simulink model "HydrogenRefuelingStation_Param"  (R2023b)
settings: Solver=VariableStepAuto  StartTime=0.0  StopTime=finSimulation  RelTol=1e-3  AbsTol=1e-3
PreLoadFcn:
  | load hydrogen_properties.mat
  | load silicone_fluid_properties.mat
  | 
  | p_storage = 200; % [bar]
  | p_vehicle_init = 100; % [bar]
  | T_env = 25; % [degC]
  | T_fluid = -60; % [degC]
  | 
  | V_vehicle = 172; % [l]
  | 
  | tube_D = 0.04; % [m]
  | hose_D = 0.0064; % [m]
  | pipe_D = 0.1; % [m]
  | 
  | num_buffer = 2;
  | 
  | intercooler_num_tubes = 25;
  | intercooler_tube_D = 0.008; % [m]
  | intercooler_shell_D = 0.1; % [m]
  | intercooler_L = 2; % [m]
  | 
  | precooler_tube_W = 0.001; % [m]
  | precooler_num_tubes = 50*25;
  | precooler_L = 1; % [m]
values from neighbouring files (symbols this model uses):
  EngDemandTime = 3000    [launch.m]
  EngThrottle = 1    [launch.m]
  ext_bufferEng_D = 0.025    [System_Parameters.m]
  ext_Manifold_D = 0.007    [System_Parameters.m]
  ext_vehTank_D = 0.25    [System_Parameters.m]
  in_bufferEng_D = 0.0064    [System_Parameters.m]
  in_Eng_D = 0.0064    [System_Parameters.m]
  in_Man_D = 0.0064    [System_Parameters.m]
  inOut_vehTank_D = 0.0064    [System_Parameters.m]
  int_bufferEng_D = 0.024    [System_Parameters.m]
  int_Manifold_D = 0.0064    [System_Parameters.m]
  int_vehTank_D = 0.22    [System_Parameters.m]
  L_bufferEng = 1    [System_Parameters.m]
  L_Manifold = 1    [System_Parameters.m]
  L_vehTank = 2    [System_Parameters.m]
  MV_D = 0.0064    [System_Parameters.m]
  out_bufferEng_D = 0.0064/2    (= 0.0032)    [System_Parameters.m]
  out_Eng_D = 0.0064    [System_Parameters.m]
  out_Man_D = 0.0064    [System_Parameters.m]
  Pipe_ConnMan_D = 0.0064    [System_Parameters.m]
  Pipe_ManPR_D = 0.0064    [System_Parameters.m]
  Pipe_ManTank_D = 0.0064    [System_Parameters.m]
  Pipe_PRBuffer_D = 0.0064    [System_Parameters.m]
  redn_PR_D = 0.0064    [System_Parameters.m]
  redn_PR_setP = 160    [System_Parameters.m]
  relief_PR_D = 0.0064    [System_Parameters.m]
  relief_vehTank_D = 0.0064    [System_Parameters.m]
  silicone_fluid =     [silicone_fluid_properties.mat]
  statConn_D = 0.0064    [System_Parameters.m]
  stationTrigger_Time = 2400    [System_Parameters.m]
  SV_D = 0.0064    [System_Parameters.m]
  tank_Man_D = 0.0064    [System_Parameters.m]
  TempCont_vehTank_D = 0.0064    [System_Parameters.m]
  vehConn_D = 0.0064    [System_Parameters.m]
  WP_high = 700    [System_Parameters.m]
libraries: fl_lib x128, nesl_utility x60, SimscapeFluids_lib x41, slpidlib x4
(part 4 of 6)

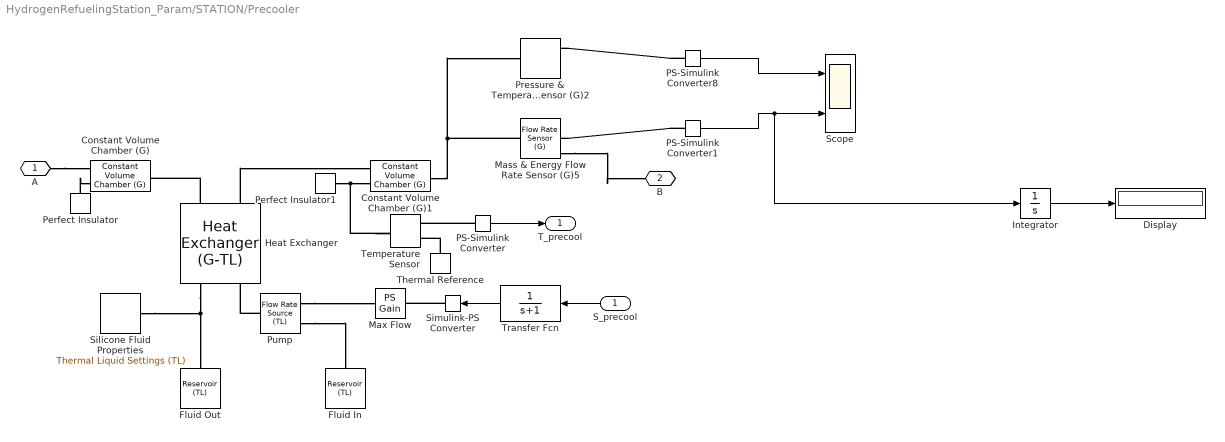
== system HydrogenRefuelingStation_Param/STATION/Precooler ==
  S_precool : Inport
  Constant Volume Chamber (G) : fl_lib/Gas/Elements/Constant Volume Chamber (G)  volume=0.1 l  num_ports=foundation.enum.num_ports.two  area_A=pi*tube_D^2/4 m^2  area_B=precooler_num_tubes * precooler_tube_W^2 m^2  area_C=0.01 m^2  area_D=0.01 m^2  p_I_specify=on  p_I_priority=High  p_I=p_vehTank_init bar  p_I_nominal_specify=off  p_I_nominal_unit=MPa  p_I_nominal_value=1  T_I_specify=on  T_I_priority=High  T_I=T_env degC  T_I_nominal_specify=off  T_I_nominal_unit=K  T_I_nominal_value=1  rho_I_specify=off  rho_I_priority=None  rho_I=1.2 kg/m^3  rho_I_nominal_specify=off  rho_I_nominal_unit=kg/m^3  rho_I_nominal_value=1
      settings: InternalSimscapePortConfiguration="{\"Bottom\":[],\"Left\":[{\"id\":\"A\",\"label\":\"A\",\"type\":\"foundation.gas.gas\"},{\"id\":\"H\",\"label\":\"H\",\"type\":\"foundation.thermal.thermal\"}],\"Right\":[{\"id\":\"B\",\"label\":\"B\",\"type\":\"foundation.gas.gas\"}],\"Top\":[]}"
  Constant Volume Chamber (G)1 : fl_lib/Gas/Elements/Constant Volume Chamber (G)  volume=0.1 l  num_ports=foundation.enum.num_ports.two  area_A=precooler_num_tubes * precooler_tube_W^2 m^2  area_B=pi*hose_D^2/4 m^2  area_C=0.01 m^2  area_D=0.01 m^2  p_I_specify=on  p_I_priority=High  p_I=p_vehTank_init bar  p_I_nominal_specify=off  p_I_nominal_unit=MPa  p_I_nominal_value=1  T_I_specify=on  T_I_priority=High  T_I=T_env degC  T_I_nominal_specify=off  T_I_nominal_unit=K  T_I_nominal_value=1  rho_I_specify=off  rho_I_priority=None  rho_I=1.2 kg/m^3  rho_I_nominal_specify=off  rho_I_nominal_unit=kg/m^3  rho_I_nominal_value=1
      settings: InternalSimscapePortConfiguration="{\"Bottom\":[],\"Left\":[{\"id\":\"A\",\"label\":\"A\",\"type\":\"foundation.gas.gas\"},{\"id\":\"H\",\"label\":\"H\",\"type\":\"foundation.thermal.thermal\"}],\"Right\":[{\"id\":\"B\",\"label\":\"B\",\"type\":\"foundation.gas.gas\"}],\"Top\":[]}"
  Display : Display
  Fluid In : fl_lib/Thermal Liquid/Elements/Reservoir (TL)  pressure_spec=foundation.enum.pressure_spec.atmospheric  reservoir_pressure=0.101325 MPa  reservoir_temperature=T_fluid degC  area=pi*pipe_D^2/4 m^2
  Fluid Out : fl_lib/Thermal Liquid/Elements/Reservoir (TL)  pressure_spec=foundation.enum.pressure_spec.atmospheric  reservoir_pressure=0.101325 MPa  reservoir_temperature=T_fluid degC  area=pi*pipe_D^2/4 m^2
  Heat Exchanger : SimscapeFluids_lib/Fluid Network Interfaces/Heat Exchangers/Heat Exchanger (G-TL)  hex_type=fluids.interfaces.enum.flow_arrangement_spec.parallel_counter  shell_num=1  cross_type=fluids.interfaces.enum.cross_flow_heat_exchanger_G_TL_spec.mixed_mixed  NTU_TLU=[.5, 1, 2, 3, 4, 5]  CR_TLU=[0, .25, .5, .75, 1]  eff_TLU=[.3, .3, .3, .3, .3; .6, .55, .5, .47, .43; .85, .76, .68, .61, .55; .94, .83, .72, .65, .58; .98, .86, .75, .66, .58; .99, .86, .75, .66, .58]  wall_thermal_dynamics=simscape.enum.onoff.off  thermal_mass_wall=447 J/K  R_wall=0 K/W  min_flow_area_1=precooler_num_tubes * precooler_tube_W^2 m^2  Dh_press_1=precooler_tube_W m  gas_volume_1=precooler_num_tubes * precooler_tube_W^2 * precooler_L m^3  Re_lam_1=2000  Re_tur_1=4000  pressure_loss_spec_1=fluids.interfaces.enum.pressure_loss_spec.tube_correlation  pressure_loss_coeff_1=0.1  length_press_1=precooler_L m  length_add_1=0.3 m  roughness_1=15e-6 m  Re_friction_TLU_1=[400, 1000, 1500, 3000, 4000, 6000, 10000, 20000, 40000, 60000, 100000, 100000000]  friction_factor_TLU_1=[.264, .112, .071, .0417, .0387, .0268, .025, .0232, .0226, .022, .0214, .0214]  shape_factor_1=56.92  Re_Euler_TLU_1=[50, 500, 1000, 2000]  Euler_TLU_1=[4.4505, .6864, .4791, .3755]  heat_transfer_spec_1=fluids.interfaces.enum.heat_transfer_spec.tube_correlation  heat_transfer_area_1=precooler_num_tubes * 4 * precooler_tube_W * precooler_L m^2  heat_coeff_1=100 W/(K*m^2)  length_heat_1=precooler_L m  Nu_lam_1=2.98  Re_Colburn_TLU_1=[100, 150, 1000]  Colburn_factor_TLU_1=[.019, .013, .002]  Re_Nu_TLU_1=[100, 150, 1000]  Pr_Nu_TLU_1=[1, 10]  Nu_TLU_1=[3.72, 4.21; 3.75, 4.44; 4.21, 7.15]  fouling_factor_1=0 K*m^2/W  mdot_threshold_1=1e-6 kg/s  min_heat_coeff_1=5 W/(K*m^2)  min_flow_area_2=precooler_num_tubes * precooler_tube_W^2 m^2  Dh_press_2="precooler_tube_W  m"  liquid_volume_2=precooler_num_tubes * precooler_tube_W^2 * precooler_L m^3  Re_lam_2=2000  Re_tur_2=4000  pressure_loss_spec_2=fluids.interfaces.enum.pressure_loss_spec.tube_correlation  pressure_loss_coeff_2=0.1  length_press_2=precooler_L m  length_add_2=0.3 m  roughness_2=15e-6 m  Re_friction_TLU_2=[400, 1000, 1500, 3000, 4000, 6000, 10000, 20000, 40000, 60000, 100000, 100000000]  friction_factor_TLU_2=[.264, .112, .071, .0417, .0387, .0268, .025, .0232, .0226, .022, .0214, .0214]  shape_factor_2=56.92  Re_Euler_TLU_2=[50, 500, 1000, 2000]  Euler_TLU_2=[4.4505, .6864, .4791, .3755]  heat_transfer_spec_2=fluids.interfaces.enum.heat_transfer_spec.tube_correlation  heat_transfer_area_2=precooler_num_tubes * 4 * precooler_tube_W * precooler_L m^2  heat_coeff_2=100 W/(K*m^2)  length_heat_2=precooler_L m  Nu_lam_2=2.98  Re_Colburn_TLU_2=[100, 150, 1000]  Colburn_factor_TLU_2=[.019, .013, .002]  Re_Nu_TLU_2=[100, 150, 1000]  Pr_Nu_TLU_2=[1, 10]  Nu_TLU_2=[3.72, 4.21; 3.75, 4.44; 4.21, 7.15]  fouling_factor_2=0 K*m^2/W  min_heat_coeff_2=5 W/(K*m^2)  T0_1=T_env degC  p0_1=p_vehTank_init bar  dynamic_compressibility_2=simscape.enum.onoff.on  T0_2=T_fluid degC  p0_2=0.101325 MPa  mdot1_TLU=[.3, .5, .6, .7, 1, 1.4, 1.9, 2.3] kg/s  mdot2_TLU=[.3, .5, 1, 1.3, 1.7, 2, 2.6, 3.3] kg/s  SD_TLU=[.324, .3533, .404, .4253, .4333, .4373, .4453, .4533; .3813, .424, .496, .5307, .544, .5547, .5693, .5787; .4267, .4827, .5813, .6173, .6413, .6573, .672, .6827; .4613, .528, .64, .6987, .7267, .7467, .7707, .7853; .5533, .6467, .8227, .928, .9853, 1.0187, 1.0653, 1.0973; .58, .688, .8853, 1.0147, 1.08, 1.124, 1.176, 1.2147; .624, .7467, .992, 1.148, 1.244, 1.304, 1.3773, 1.4267; .656, .7907, 1.0667, 1.26, 1.376, 1.452, 1.548, 1.612] kW/K  Q_check=fluids.interfaces.enum.SD_max_check.warning  mdot_dp_TLU_1=[.3, .5, 1, 1.5, 2, 2.5] kg/s  p_diff_TLU_1=[3, 5, 10, 25, 35, 50] * 1e-3 MPa  T_ref_in_1=293.15 K  p_ref_in_1=0.101325 MPa  area_1=0.01 m^2  mdot_dp_TLU_2=[.3, .5, 1, 1.5, 2, 2.5] kg/s  p_diff_TLU_2=[3, 5, 10, 25, 35, 50] * 1e-3 MPa  T_ref_in_2=293.15 K  p_ref_in_2=0.101325 MPa  mdot_threshold_2=1e-3 kg/s  area_2=0.01 m^2
      settings: InternalSimscapePortConfiguration="{\"Bottom\":[],\"Left\":[{\"id\":\"A1\",\"label\":\"A1\",\"type\":\"foundation.gas.gas\"},{\"id\":\"B1\",\"label\":\"B1\",\"type\":\"foundation.gas.gas\"}],\"Right\":[{\"id\":\"A2\",\"label\":\"A2\",\"type\":\"foundation.thermal_liquid.thermal_liquid\"},{\"id\":\"B2\",\"label\":\"B2\",\"type\":\"foundation.thermal_liquid.thermal_liquid\"}],\"Top\":[]}"
  Integrator : Integrator
  Mass & Energy Flow Rate Sensor (G)5 : fl_lib/Gas/Sensors/Flow Rate Sensor (G)  mass_flow_measure=true  volumetric_flow_measure=false  volumetric_flow_conditions=foundation.enum.volumetric_flow_conditions.actual  p_std=0.101325 MPa  T_std=20 degC  energy_flow_measure=true
      settings: InternalSimscapePortConfiguration="{\"Bottom\":[{\"id\":\"PHI\",\"label\":\"φ\",\"type\":\"output\"}],\"Left\":[{\"id\":\"A\",\"label\":\"A\",\"type\":\"foundation.gas.gas\"}],\"Right\":[{\"id\":\"B\",\"label\":\"B\",\"type\":\"foundation.gas.gas\"},{\"id\":\"M\",\"label\":\"M\",\"type\":\"output\"}],\"Top\":[]}"
  Max Flow : fl_lib/Physical Signals/Functions/PS Gain  gain=1 kg/s
  PS-Simulink Converter : nesl_utility/PS-Simulink Converter  PhysicalDomain=network_engine_domain  SubClassName=ps_output  LeftPortType=input  RightPortType=output  PseudoPeriodic=off  Frequencies=[]  VectorFormat=inherit  Unit=degC  AffineConversion=on
  PS-Simulink Converter1 : nesl_utility/PS-Simulink Converter  PhysicalDomain=network_engine_domain  SubClassName=ps_output  LeftPortType=input  RightPortType=output  PseudoPeriodic=off  Frequencies=[]  VectorFormat=inherit  Unit=kg/s  AffineConversion=off
  PS-Simulink Converter8 : nesl_utility/PS-Simulink Converter  PhysicalDomain=network_engine_domain  SubClassName=ps_output  LeftPortType=input  RightPortType=output  PseudoPeriodic=off  Frequencies=[]  VectorFormat=inherit  Unit=bar  AffineConversion=off
  Perfect Insulator : fl_lib/Thermal/Thermal Elements/Perfect Insulator  T_specify=off  T_priority=None  T=293.15 K  T_nominal_specify=off  T_nominal_unit=K  T_nominal_value=1
  Perfect Insulator1 : fl_lib/Thermal/Thermal Elements/Perfect Insulator  T_specify=off  T_priority=None  T=293.15 K  T_nominal_specify=off  T_nominal_unit=K  T_nominal_value=1
  Pressure & Temperature Sensor (G)2 : fl_lib/Gas/Sensors/Pressure & Temperature Sensor (G)  reference=foundation.enum.MeasurementReference.absolute  pressure=true  pressure_spec=foundation.enum.PressureMeasementSpec.Absolute  temperature=true
      settings: InternalSimscapePortConfiguration="{\"Bottom\":[{\"id\":\"T\",\"label\":\"T\",\"type\":\"output\"}],\"Left\":[{\"id\":\"A\",\"label\":\"A\",\"type\":\"foundation.gas.gas\"}],\"Right\":[{\"id\":\"Pa\",\"label\":\"Pa\",\"type\":\"output\"}],\"Top\":[]}"
  Pump : fl_lib/Thermal Liquid/Sources/Flow Rate Source (TL)  source_type=foundation.enum.constant_controlled.controlled  flow_type=foundation.enum.mass_volumetric_flow.mass  mass_flow=0 kg/s  volumetric_flow=0 m^3/s  power_spec=foundation.enum.power_spec.isentropic  area=pi*pipe_D^2/4 m^2
  Scope : Scope  NumInputPorts=2
  Silicone Fluid Properties : fl_lib/Thermal Liquid/Utilities/Thermal Liquid Settings (TL)  table_dimensions=foundation.enum.table_dimensions_TL.one_dimensional  T_TLU=silicone_fluid.T K  p_TLU=[0.01, 0.1, 5 : 5 : 50] MPa  p_atm=0.101325 MPa  pT_region_flag=foundation.enum.pT_region_TL.min_max  T_min=273.16 K  T_max=363.16 K  p_min=0.05 MPa  p_max=50 MPa  T_min_1D=silicone_fluid.T(1) K  T_max_1D=silicone_fluid.T(end) K  p_min_1D=0.05 MPa  p_max_1D=50 MPa  pT_validity_TLU=[1, 1, 1, 1, 1, 1, 1, 1, 1, 1, 1, 1; 1, 1, 1, 1, 1, 1, 1, 1, 1, 1, 1, 1; 1, 1, 1, 1, 1, 1, 1, 1, 1, 1, 1, 1; 1, 1, 1, 1, 1, 1, 1, 1, 1, 1, 1, 1; 1, 1, 1, 1, 1, 1, 1, 1, 1, 1, 1, 1; 0, 1, 1, 1, 1, 1, 1, 1, 1, 1, 1, 1; 0, 1, 1, 1, 1, 1, 1, 1, 1, 1, 1, 1; 0, 1, 1, 1, 1, 1, 1, 1, 1, 1, 1, 1; 0, 1, 1, 1, 1, 1, 1, 1, 1, 1, 1, 1; 0, 1, 1, 1, 1, 1, 1, 1, 1, 1, 1, 1; 0, 0, 1, 1, 1, 1, 1, 1, 1, 1, 1, 1]  properties_range_check=simscape.enum.assert.action.error  rho_parameterization_2D=foundation.enum.rho_parameterization_2D.rho_beta_alpha  rho_parameterization_1D=foundation.enum.rho_parameterization_1D.rho_vector  rho_TLU=[999.7973, 999.8431, 1002.3216, 1004.8218, 1007.293, 1009.7358, 1012.1506, 1014.5379, 1016.8979, 1019.2311, 1021.538, 1023.8188; 999.6579, 999.7009, 1002.0303, 1004.382, 1006.7084, 1009.0101, 1011.2874, 1013.5407, 1015.7703, 1017.9766, 1020.1599, 1022.3206; 998.1632, 998.2045, 1000.4375, 1002.6924, 1004.9239, 1007.1324, 1009.3183, 1011.4819, 1013.6236, 1015.7438, 1017.8428, 1019.921; 995.6057, 995.6458, 997.81864, 1000.0128, 1002.1841, 1004.3332, 1006.4603, 1008.566, 1010.6505, 1012.7144, 1014.758, 1016.7815; 992.1724, 992.2119, 994.35133, 996.5113, 998.6484, 1000.7633, 1002.8563, 1004.928, 1006.9788, 1009.009, 1011.0192, 1013.0097; 988.02, 988.0299, 990.15684, 992.3035, 994.4268, 996.5273, 998.6056, 1000.6622, 1002.6976, 1004.7123, 1006.7067, 1008.6813; 983.18, 983.1901, 985.3217, 987.4721, 989.5983, 991.7008, 993.7803, 995.8374, 997.8726, 999.8864, 1001.8795, 1003.8522; 977.75, 977.7583, 979.9094, 982.0783, 984.2216, 986.34, 988.4343, 990.505, 992.5529, 994.5786, 996.5825, 998.5654; 971.77, 971.7836, 973.96734, 976.1678, 978.3409, 980.4876, 982.6087, 984.7049, 986.7768, 988.8254, 990.8511, 992.8545; 965.26, 965.3023, 967.53107, 969.7753, 971.9901, 974.1764, 976.3354, 978.4676, 980.5741, 982.6556, 984.7129, 986.7465; 958.62, 958.6315, 960.627, 962.9267, 965.1944, 967.4314, 969.6387, 971.8173, 973.9681, 976.0921, 978.19, 980.2628] kg/m^3  beta_TLU=[1.9649, 1.9654, 1.9929, 2.0213, 2.0499, 2.0787, 2.1078, 2.1372, 2.1668, 2.1966, 2.2268, 2.2572; 2.0913, 2.0918, 2.1191, 2.1471, 2.1752, 2.2036, 2.2322, 2.261, 2.2899, 2.3191, 2.3485, 2.3781; 2.1786, 2.1791, 2.2067, 2.235, 2.2634, 2.2919, 2.3206, 2.3494, 2.3784, 2.4075, 2.4367, 2.4661; 2.2332, 2.2337, 2.2619, 2.2908, 2.3197, 2.3487, 2.3778, 2.407, 2.4363, 2.4657, 2.4951, 2.5246; 2.26, 2.2605, 2.2895, 2.3191, 2.3487, 2.3784, 2.4081, 2.4378, 2.4675, 2.4973, 2.5272, 2.5571; 2.2638, 2.2638, 2.2936, 2.324, 2.3544, 2.3848, 2.4151, 2.4455, 2.4758, 2.5062, 2.5365, 2.5669; 2.2472, 2.2472, 2.2779, 2.3092, 2.3403, 2.3715, 2.4025, 2.4336, 2.4646, 2.4955, 2.5264, 2.5573; 2.214, 2.214, 2.2455, 2.2776, 2.3096, 2.3415, 2.3733, 2.405, 2.4367, 2.4683, 2.4998, 2.5313; 2.1668, 2.1668, 2.1992, 2.2321, 2.2649, 2.2976, 2.3301, 2.3626, 2.3949, 2.4272, 2.4593, 2.4914; 2.1081, 2.1081, 2.1413, 2.175, 2.2086, 2.2421, 2.2754, 2.3085, 2.3415, 2.3744, 2.4072, 2.4399; 2.0494, 2.0494, 2.0739, 2.1084, 2.1428, 2.177, 2.211, 2.2449, 2.2786, 2.3121, 2.3455, 2.3788] GPa  alpha_TLU=1e-4 * [-.679, -.676, -.49, -.307, -.13, .041, .206, .365, .519, .668, .811, .949; .878, .881, .998, 1.114, 1.227, 1.337, 1.445, 1.549, 1.651, 1.75, 1.846, 1.939; 2.068, 2.069, 2.141, 2.213, 2.283, 2.352, 2.42, 2.486, 2.551, 2.614, 2.676, 2.736; 3.034, 3.035, 3.074, 3.113, 3.152, 3.191, 3.229, 3.267, 3.305, 3.341, 3.377, 3.413; 3.855, 3.856, 3.87, 3.884, 3.899, 3.914, 3.93, 3.946, 3.961, 3.977, 3.993, 4.009; 4.578, 4.578, 4.572, 4.566, 4.562, 4.558, 4.555, 4.552, 4.55, 4.549, 4.548, 4.547; 5.233, 5.233, 5.209, 5.186, 5.165, 5.144, 5.125, 5.107, 5.09, 5.074, 5.059, 5.045; 5.84, 5.84, 5.801, 5.762, 5.725, 5.691, 5.657, 5.625, 5.595, 5.566, 5.538, 5.512; 6.414, 6.414, 6.36, 6.307, 6.256, 6.208, 6.161, 6.117, 6.074, 6.033, 5.994, 5.956; 6.967, 6.967, 6.898, 6.831, 6.766, 6.705, 6.646, 6.589, 6.535, 6.482, 6.432, 6.384; 7.519, 7.519, 7.423, 7.342, 7.264, 7.189, 7.118, 7.049, 6.983, 6.92, 6.859, 6.8] 1/K  rho_TLU_2=[999.7973, 999.8431, 1002.3216, 1004.8218, 1007.293, 1009.7358, 1012.1506, 1014.5379, 1016.8979, 1019.2311, 1021.538, 1023.8188; 999.6579, 999.7009, 1002.0303, 1004.382, 1006.7084, 1009.0101, 1011.2874, 1013.5407, 1015.7703, 1017.9766, 1020.1599, 1022.3206; 998.1632, 998.2045, 1000.4375, 1002.6924, 1004.9239, 1007.1324, 1009.3183, 1011.4819, 1013.6236, 1015.7438, 1017.8428, 1019.921; 995.6057, 995.6458, 997.81864, 1000.0128, 1002.1841, 1004.3332, 1006.4603, 1008.566, 1010.6505, 1012.7144, 1014.758, 1016.7815; 992.1724, 992.2119, 994.35133, 996.5113, 998.6484, 1000.7633, 1002.8563, 1004.928, 1006.9788, 1009.009, 1011.0192, 1013.0097; 988.02, 988.0299, 990.15684, 992.3035, 994.4268, 996.5273, 998.6056, 1000.6622, 1002.6976, 1004.7123, 1006.7067, 1008.6813; 983.18, 983.1901, 985.3217, 987.4721, 989.5983, 991.7008, 993.7803, 995.8374, 997.8726, 999.8864, 1001.8795, 1003.8522; 977.75, 977.7583, 979.9094, 982.0783, 984.2216, 986.34, 988.4343, 990.505, 992.5529, 994.5786, 996.5825, 998.5654; 971.77, 971.7836, 973.96734, 976.1678, 978.3409, 980.4876, 982.6087, 984.7049, 986.7768, 988.8254, 990.8511, 992.8545; 965.26, 965.3023, 967.53107, 969.7753, 971.9901, 974.1764, 976.3354, 978.4676, 980.5741, 982.6556, 984.7129, 986.7465; 958.62, 958.6315, 960.627, 962.9267, 965.1944, 967.4314, 969.6387, 971.8173, 973.9681, 976.0921, 978.19, 980.2628] kg/m^3  rho_ref_3=998.21 kg/m^3  T_ref_3=293.16 K  p_ref_3=0.101325 MPa  beta_const_3=2.1791 GPa  alpha_const_3=2.0691e-4 1/K  rho_TLU_4=silicone_fluid.rho kg/m^3  beta_const_4=silicone_fluid.beta GPa  p_ref_4=0.101325 MPa  rho_ref_5=998.21 kg/m^3  T_ref_5=293.16 K  p_ref_5=0.101325 MPa  beta_const_5=2.1791 GPa  alpha_const_5=2.0691e-4 1/K  u_parameterization_2D=foundation.enum.u_parameterization_2D.u_cp  u_parameterization_1D=foundation.enum.u_parameterization_1D.cp  u_TLU=[.0002, .0018, .086, .1588, .219, .267, .3034, .3288, .3436, .3483, .3435, .3294; 42.062, 42.06, 41.935, 41.804, 41.668, 41.527, 41.382, 41.233, 41.081, 40.924, 40.763, 40.599; 83.953, 83.948, 83.651, 83.349, 83.049, 82.749, 82.451, 82.153, 81.856, 81.56, 81.265, 80.971; 125.77, 125.76, 125.31, 124.86, 124.41, 123.97, 123.53, 123.1, 122.68, 122.25, 121.84, 121.42; 167.57, 167.56, 166.96, 166.37, 165.79, 165.21, 164.65, 164.09, 163.54, 163, 162.46, 161.94; 209.36, 209.36, 208.63, 207.9, 207.19, 206.48, 205.79, 205.11, 204.45, 203.79, 203.14, 202.5; 251.19, 251.19, 250.33, 249.47, 248.62, 247.79, 246.98, 246.18, 245.39, 244.62, 243.86, 243.12; 293.06, 293.06, 292.07, 291.07, 290.1, 289.14, 288.2, 287.28, 286.38, 285.49, 284.62, 283.77; 334.99, 334.99, 333.86, 332.73, 331.63, 330.54, 329.48, 328.44, 327.41, 326.41, 325.43, 324.46; 377, 377, 375.73, 374.46, 373.22, 372, 370.81, 369.64, 368.5, 367.38, 366.27, 365.19; 419.01, 419.01, 417.69, 416.27, 414.89, 413.54, 412.21, 410.91, 409.64, 408.4, 407.17, 405.98] kJ/kg  cp_TLU=[4.2199, 4.2194, 4.1957, 4.1726, 4.1508, 4.13, 4.1103, 4.0916, 4.0738, 4.0569, 4.0408, 4.0254; 4.1955, 4.1951, 4.1769, 4.1592, 4.1422, 4.1259, 4.1103, 4.0954, 4.0812, 4.0676, 4.0545, 4.0421; 4.1843, 4.184, 4.169, 4.1543, 4.1401, 4.1264, 4.1133, 4.1007, 4.0885, 4.0768, 4.0656, 4.0548; 4.1801, 4.1798, 4.1667, 4.1538, 4.1413, 4.1293, 4.1177, 4.1064, 4.0956, 4.0851, 4.075, 4.0653; 4.1796, 4.1794, 4.1675, 4.1558, 4.1444, 4.1334, 4.1227, 4.1123, 4.1023, 4.0926, 4.0832, 4.0741; 4.1813, 4.1813, 4.1702, 4.1592, 4.1484, 4.138, 4.1279, 4.1181, 4.1086, 4.0993, 4.0903, 4.0816; 4.185, 4.185, 4.1742, 4.1636, 4.1532, 4.1432, 4.1334, 4.1239, 4.1146, 4.1056, 4.0969, 4.0884; 4.1901, 4.1901, 4.1795, 4.169, 4.1588, 4.1489, 4.1393, 4.1299, 4.1207, 4.1118, 4.1032, 4.0947; 4.1968, 4.1968, 4.1862, 4.1757, 4.1655, 4.1555, 4.1458, 4.1364, 4.1273, 4.1183, 4.1096, 4.1012; 4.2052, 4.2052, 4.1944, 4.1837, 4.1733, 4.1632, 4.1534, 4.1438, 4.1345, 4.1255, 4.1166, 4.108; 4.2136, 4.2136, 4.2045, 4.1935, 4.1828, 4.1724, 4.1623, 4.1524, 4.1429, 4.1335, 4.1245, 4.1157] kJ/(K*kg)  u_TLU_2=[.0002, .0018, .086, .1588, .219, .267, .3034, .3288, .3436, .3483, .3435, .3294; 42.062, 42.06, 41.935, 41.804, 41.668, 41.527, 41.382, 41.233, 41.081, 40.924, 40.763, 40.599; 83.953, 83.948, 83.651, 83.349, 83.049, 82.749, 82.451, 82.153, 81.856, 81.56, 81.265, 80.971; 125.77, 125.76, 125.31, 124.86, 124.41, 123.97, 123.53, 123.1, 122.68, 122.25, 121.84, 121.42; 167.57, 167.56, 166.96, 166.37, 165.79, 165.21, 164.65, 164.09, 163.54, 163, 162.46, 161.94; 209.36, 209.36, 208.63, 207.9, 207.19, 206.48, 205.79, 205.11, 204.45, 203.79, 203.14, 202.5; 251.19, 251.19, 250.33, 249.47, 248.62, 247.79, 246.98, 246.18, 245.39, 244.62, 243.86, 243.12; 293.06, 293.06, 292.07, 291.07, 290.1, 289.14, 288.2, 287.28, 286.38, 285.49, 284.62, 283.77; 334.99, 334.99, 333.86, 332.73, 331.63, 330.54, 329.48, 328.44, 327.41, 326.41, 325.43, 324.46; 377, 377, 375.73, 374.46, 373.22, 372, 370.81, 369.64, 368.5, 367.38, 366.27, 365.19; 419.01, 419.01, 417.69, 416.27, 414.89, 413.54, 412.21, 410.91, 409.64, 408.4, 407.17, 405.98] kJ/kg  cp_TLU_3=[4.2199, 4.2194, 4.1957, 4.1726, 4.1508, 4.13, 4.1103, 4.0916, 4.0738, 4.0569, 4.0408, 4.0254; 4.1955, 4.1951, 4.1769, 4.1592, 4.1422, 4.1259, 4.1103, 4.0954, 4.0812, 4.0676, 4.0545, 4.0421; 4.1843, 4.184, 4.169, 4.1543, 4.1401, 4.1264, 4.1133, 4.1007, 4.0885, 4.0768, 4.0656, 4.0548; 4.1801, 4.1798, 4.1667, 4.1538, 4.1413, 4.1293, 4.1177, 4.1064, 4.0956, 4.0851, 4.075, 4.0653; 4.1796, 4.1794, 4.1675, 4.1558, 4.1444, 4.1334, 4.1227, 4.1123, 4.1023, 4.0926, 4.0832, 4.0741; 4.1813, 4.1813, 4.1702, 4.1592, 4.1484, 4.138, 4.1279, 4.1181, 4.1086, 4.0993, 4.0903, 4.0816; 4.185, 4.185, 4.1742, 4.1636, 4.1532, 4.1432, 4.1334, 4.1239, 4.1146, 4.1056, 4.0969, 4.0884; 4.1901, 4.1901, 4.1795, 4.169, 4.1588, 4.1489, 4.1393, 4.1299, 4.1207, 4.1118, 4.1032, 4.0947; 4.1968, 4.1968, 4.1862, 4.1757, 4.1655, 4.1555, 4.1458, 4.1364, 4.1273, 4.1183, 4.1096, 4.1012; 4.2052, 4.2052, 4.1944, 4.1837, 4.1733, 4.1632, 4.1534, 4.1438, 4.1345, 4.1255, 4.1166, 4.108; 4.2136, 4.2136, 4.2045, 4.1935, 4.1828, 4.1724, 4.1623, 4.1524, 4.1429, 4.1335, 4.1245, 4.1157] kJ/(K*kg)  u_TLU_4=[.0018; 42.06; 83.948; 125.76; 167.56; 209.36; 251.19; 293.06; 334.99; 377; 418.01] kJ/kg  cp_TLU_5=silicone_fluid.cp kJ/(K*kg)  nu_TLU=[1.7917, 1.7914, 1.7763, 1.7615, 1.7473, 1.7338, 1.7208, 1.7085, 1.6967, 1.6854, 1.6747, 1.6645; 1.3061, 1.3059, 1.2986, 1.2914, 1.2845, 1.2779, 1.2716, 1.2656, 1.2598, 1.2543, 1.2491, 1.2441; 1.0032, 1.0032, .9995, .9959, .9924, .9891, .9859, .9829, .9801, .9774, .9748, .9724; .8006, .8005, .7987, .797, .7953, .7937, .7922, .7908, .7894, .7881, .787, .7859; .6577, .6577, .657, .6562, .6555, .6548, .6543, .6537, .6532, .6528, .6523, .652; .553, .553, .5529, .5527, .5526, .5525, .5524, .5524, .5524, .5524, .5524, .5525; .4739, .4739, .4741, .4743, .4745, .4747, .475, .4753, .4755, .4758, .4762, .4765; .4127, .4127, .4131, .4135, .4139, .4143, .4148, .4152, .4157, .4162, .4167, .4172; .3643, .3643, .3648, .3654, .3659, .3665, .367, .3676, .3682, .3688, .3694, .37; .3254, .3254, .3261, .3267, .3273, .328, .3286, .3293, .3299, .3306, .3312, .3319; .2866, .2866, .2945, .2952, .2959, .2965, .2972, .2979, .2986, .2993, .3, .3007] mm^2/s  nu_TLU_2=silicone_fluid.nu mm^2/s  k_TLU=[561.04, 561.09, 563.8, 566.56, 569.32, 572.08, 574.82, 577.54, 580.24, 582.92, 585.57, 588.18; 580.02, 580.07, 582.45, 584.88, 587.32, 589.75, 592.18, 594.61, 597.02, 599.42, 601.8, 604.16; 598.44, 598.48, 600.73, 603.03, 605.33, 607.64, 609.94, 612.24, 614.54, 616.82, 619.1, 621.36; 615.48, 615.52, 617.73, 620, 622.26, 624.54, 626.81, 629.07, 631.34, 633.6, 635.85, 638.09; 630.6, 630.64, 632.87, 635.15, 637.44, 639.72, 642.01, 644.29, 646.57, 648.84, 651.11, 653.36; 643.61, 643.61, 645.88, 648.21, 650.53, 652.86, 655.18, 657.51, 659.82, 662.14, 664.44, 666.74; 654.39, 654.39, 656.73, 659.12, 661.5, 663.89, 666.27, 668.65, 671.02, 673.38, 675.74, 678.09; 663.13, 663.13, 665.54, 668, 670.46, 672.91, 675.36, 677.8, 680.24, 682.67, 685.09, 687.5; 670.02, 670.02, 672.51, 675.05, 677.59, 680.12, 682.64, 685.16, 687.67, 690.17, 692.66, 695.14; 675.27, 675.27, 677.85, 680.48, 683.11, 685.73, 688.34, 690.94, 693.53, 696.11, 698.68, 701.24; 680.52, 680.52, 681.77, 684.5, 687.22, 689.94, 692.64, 695.34, 698.02, 700.69, 703.35, 706] mW/(K*m)  k_TLU_2=silicone_fluid.k mW/(K*m)
  Simulink-PS Converter : nesl_utility/Simulink-PS Converter  PhysicalDomain=network_engine_domain  SubClassName=ps_input  LeftPortType=input  RightPortType=output  PseudoPeriodic=off  Frequencies=[]  NoiseDistribution=none  NoiseParameters=[]  Unit=1  AffineConversion=off  FilteringAndDerivatives=provide  SimscapeFilterOrder=1  InputFilterTimeConstant=0.001  UdotUserProvided=0
  Temperature Sensor : fl_lib/Thermal/Thermal Sensors/Temperature Sensor  temperature_measure=foundation.enum.MeasurementReference.difference
  Thermal Reference : fl_lib/Thermal/Thermal Elements/Thermal Reference
  Transfer Fcn : TransferFcn  Denominator=[1 1]
  A : PMIOPort  Side=Left
  B : PMIOPort  Port=2  Side=Right
  T_precool : Outport
  wires:
  Transfer Fcn/1 -> Simulink-PS Converter/1
  S_precool/1 -> Transfer Fcn/1
  PS-Simulink Converter/1 -> T_precool/1
  PS-Simulink Converter8/1 -> Scope/1
  PS-Simulink Converter1/1 -> Integrator/1, Scope/2
  Integrator/1 -> Display/1
  connections:
  A/RConn1 -- Constant Volume Chamber (G)/LConn1
  Heat Exchanger/LConn1 -- Constant Volume Chamber (G)/RConn1
  Heat Exchanger/LConn2 -- Constant Volume Chamber (G)1/LConn1
  Constant Volume Chamber (G)1/RConn1 -- Pressure & Temperature Sensor (G)2/LConn1 -- Mass & Energy Flow Rate Sensor (G)5/LConn1
  Perfect Insulator/LConn1 -- Constant Volume Chamber (G)/LConn2
  Perfect Insulator1/LConn1 -- Constant Volume Chamber (G)1/LConn2 -- Temperature Sensor/LConn1
  Silicone Fluid Properties/RConn1 -- Heat Exchanger/RConn1 -- Fluid Out/LConn1
  Pump/LConn1 -- Fluid In/LConn1
  Pump/LConn2 -- Max Flow/RConn1
  Pump/RConn1 -- Heat Exchanger/RConn2
  Simulink-PS Converter/RConn1 -- Max Flow/LConn1
  PS-Simulink Converter/LConn1 -- Temperature Sensor/RConn2
  Thermal Reference/LConn1 -- Temperature Sensor/RConn1
  PS-Simulink Converter8/LConn1 -- Pressure & Temperature Sensor (G)2/RConn1
  Mass & Energy Flow Rate Sensor (G)5/RConn1 -- B/RConn1
  PS-Simulink Converter1/LConn1 -- Mass & Energy Flow Rate Sensor (G)5/RConn2

== system HydrogenRefuelingStation_Param/STATION/Reduction Valve ==
  S_valve : Inport
  Simulink-PS Converter : nesl_utility/Simulink-PS Converter  PhysicalDomain=network_engine_domain  SubClassName=ps_input  LeftPortType=input  RightPortType=output  PseudoPeriodic=off  Frequencies=[]  NoiseDistribution=none  NoiseParameters=[]  Unit=1  AffineConversion=off  FilteringAndDerivatives=provide  SimscapeFilterOrder=1  InputFilterTimeConstant=0.001  UdotUserProvided=0
  Transfer Fcn : TransferFcn  Denominator=[1 1]
  Valve : SimscapeFluids_lib/Gas/Valves & Orifices/Orifice (G)  orifice_type=foundation.enum.constant_variable.variable  orifice_parameterization=fluids.gas.valves_orifices.enum.OrificeParameterization.Cv  opening_characteristic=fluids.gas.valves_orifices.enum.OpeningCharacteristics.Linear  Cv_constant=4  Cv_max=0.24  L_Cv_TLU=0 : 0.2 : 1  Cv_TLU=[1e-06, .8, 1.6, 2.4, 3.2, 4]  xT_Cv=0.7  Kv_constant=3.6  Kv_max=3.6  L_Kv_TLU=0 : 0.2 : 1  Kv_TLU=[1e-06, .72, 1.44, 2.16, 2.88, 3.6]  xT_Kv=0.7  C_constant=12 l/(bar*s)  B_crit_constant=0.3  C_max=12 l/(bar*s)  B_crit_linear=0.3  L_C_TLU=0 : 0.2 : 1  C_TLU=[1e-05, 2.4, 4.8, 7.2, 9.6, 12] l/(bar*s)  B_crit_TLU=0.3 * ones(1, 6)  m=0.5  T_ref_C=293.15 K  rho_ref_C=1.185 kg/m^3  orifice_area_constant=1e-4 m^2  orifice_area_max=1e-4 m^2  L_orifice_area_TLU=0 : 0.2 : 1  orifice_area_TLU=[1e-10, 2e-05, 4e-05, 6e-05, 8e-05, .0001] m^2  Cd=0.64  leakage_fraction=1e-6  smoothing_factor=0  B_lam=0.999  area=pi*tube_D^2/4 m^2
      settings: InternalSimscapePortConfiguration="{\"Bottom\":[],\"Left\":[{\"id\":\"A\",\"label\":\"A\",\"type\":\"foundation.gas.gas\"},{\"id\":\"L\",\"label\":\"L\",\"type\":\"input\"}],\"Right\":[{\"id\":\"B\",\"label\":\"B\",\"type\":\"foundation.gas.gas\"}],\"Top\":[]}"
  A : PMIOPort  Side=Left
  B : PMIOPort  Port=2  Side=Right
  wires:
  Transfer Fcn/1 -> Simulink-PS Converter/1
  S_valve/1 -> Transfer Fcn/1
  connections:
  B/RConn1 -- Valve/RConn1
  A/RConn1 -- Valve/LConn1
  Valve/LConn2 -- Simulink-PS Converter/RConn1

== system HydrogenRefuelingStation_Param/Valve Controller/Filter Derivative ==
  In1 : Inport
  Gain : Gain  Gain=1/tau
  Integrator : Integrator  InitialConditionSource=external
  Sum : Sum  Inputs=|+-
  x : Outport
  dx/dt : Outport  Port=2
  wires:
  Sum/1 -> Gain/1
  Gain/1 -> Integrator/1, dx/dt/1
  Integrator/1 -> Sum/2, x/1
  In1/1 -> Integrator/2, Sum/1

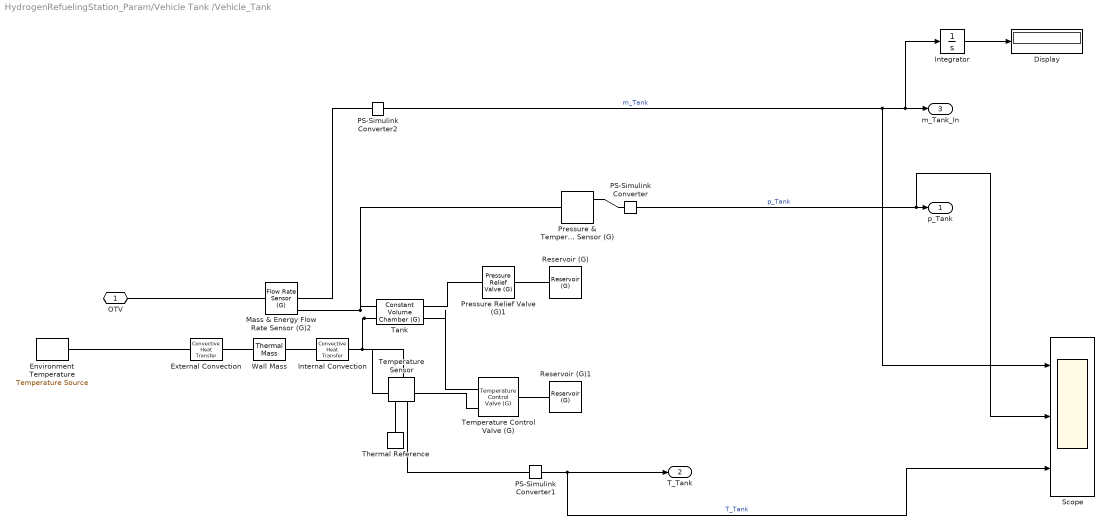
== system HydrogenRefuelingStation_Param/Vehicle Tank /Vehicle_Tank ==
  Display : Display
  Environment Temperature : fl_lib/Thermal/Thermal Sources/Temperature Source  temperature=T_env degC
  External Convection : fl_lib/Thermal/Thermal Elements/Convective Heat Transfer  thermal_type=foundation.enum.constant_variable.constant  area=2*pi*(ext_vehTank_D/2)*L_vehTank m^2  heat_tr_coeff=h_ext_vehTank W/(K*m^2)  min_heat_tr_coeff=1e-3 W/(K*m^2)  T_specify=off  T_priority=None  T=0 K  T_nominal_specify=off  T_nominal_unit=K  T_nominal_value=1  Q_specify=off  Q_priority=None  Q=0 W  Q_nominal_specify=off  Q_nominal_unit=W  Q_nominal_value=1
  Integrator : Integrator
  Internal Convection : fl_lib/Thermal/Thermal Elements/Convective Heat Transfer  thermal_type=foundation.enum.constant_variable.constant  area=2*pi*(int_vehTank_D/2)*L_vehTank m^2  heat_tr_coeff=h_int_vehTank W/(K*m^2)  min_heat_tr_coeff=1e-3 W/(K*m^2)  T_specify=off  T_priority=None  T=0 K  T_nominal_specify=off  T_nominal_unit=K  T_nominal_value=1  Q_specify=off  Q_priority=None  Q=0 W  Q_nominal_specify=off  Q_nominal_unit=W  Q_nominal_value=1
  Mass & Energy Flow Rate Sensor (G)2 : fl_lib/Gas/Sensors/Flow Rate Sensor (G)  mass_flow_measure=true  volumetric_flow_measure=false  volumetric_flow_conditions=foundation.enum.volumetric_flow_conditions.actual  p_std=0.101325 MPa  T_std=20 degC  energy_flow_measure=true
      settings: InternalSimscapePortConfiguration="{\"Bottom\":[{\"id\":\"PHI\",\"label\":\"φ\",\"type\":\"output\"}],\"Left\":[{\"id\":\"A\",\"label\":\"A\",\"type\":\"foundation.gas.gas\"}],\"Right\":[{\"id\":\"B\",\"label\":\"B\",\"type\":\"foundation.gas.gas\"},{\"id\":\"M\",\"label\":\"M\",\"type\":\"output\"}],\"Top\":[]}"
  PS-Simulink Converter : nesl_utility/PS-Simulink Converter  PhysicalDomain=network_engine_domain  SubClassName=ps_output  LeftPortType=input  RightPortType=output  PseudoPeriodic=off  Frequencies=[]  VectorFormat=inherit  Unit=bar  AffineConversion=off
  PS-Simulink Converter1 : nesl_utility/PS-Simulink Converter  PhysicalDomain=network_engine_domain  SubClassName=ps_output  LeftPortType=input  RightPortType=output  PseudoPeriodic=off  Frequencies=[]  VectorFormat=inherit  Unit=degC  AffineConversion=on
  PS-Simulink Converter2 : nesl_utility/PS-Simulink Converter  PhysicalDomain=network_engine_domain  SubClassName=ps_output  LeftPortType=input  RightPortType=output  PseudoPeriodic=off  Frequencies=[]  VectorFormat=inherit  Unit=kg/s  AffineConversion=off
  Pressure & Temperature Sensor (G) : fl_lib/Gas/Sensors/Pressure & Temperature Sensor (G)  reference=foundation.enum.MeasurementReference.absolute  pressure=true  pressure_spec=foundation.enum.PressureMeasementSpec.Absolute  temperature=true
      settings: InternalSimscapePortConfiguration="{\"Bottom\":[{\"id\":\"T\",\"label\":\"T\",\"type\":\"output\"}],\"Left\":[{\"id\":\"A\",\"label\":\"A\",\"type\":\"foundation.gas.gas\"}],\"Right\":[{\"id\":\"Pa\",\"label\":\"Pa\",\"type\":\"output\"}],\"Top\":[]}"
  Pressure Relief Valve (G)1 : SimscapeFluids_lib/Gas/Valves & Orifices/Pressure Control Valves/Pressure Relief Valve (G)  opening_pressure_spec=fluids.gas.valves_orifices.enum.PressureControlSpec.PressureA  valve_parameterization=fluids.gas.valves_orifices.enum.OrificeParameterization.Cv  opening_characteristic=fluids.gas.valves_orifices.enum.OpeningCharacteristics.Linear  p_set_differential=0 MPa  p_set_gauge=relief_vehTank_setP bar  p_range=relief_vehtank_range bar  Cv_max=4  p_diff_Cv_TLU=0.2 : 0.2 : 1.2 MPa  p_gauge_Cv_TLU=0.2 : 0.2 : 1.2 MPa  Cv_TLU=[1e-06, .8, 1.6, 2.4, 3.2, 4]  xT_Cv=0.7  Kv_max=3.6  p_diff_Kv_TLU=0.2 : 0.2 : 1.2 MPa  p_gauge_Kv_TLU=0.2 : 0.2 : 1.2 MPa  Kv_TLU=[1e-06, .72, 1.44, 2.16, 2.88, 3.6]  xT_Kv=0.7  C_max=12 l/(bar*s)  B_crit_linear=0.3  p_diff_C_TLU=0.2 : 0.2 : 1.2 MPa  p_gauge_C_TLU=0.2 : 0.2 : 1.2 MPa  C_TLU=[1e-05, 2.4, 4.8, 7.2, 9.6, 12] l/(bar*s)  B_crit_TLU=0.3 * ones(1, 6)  m=0.5  T_ref_C=293.15 K  rho_ref_C=1.185 kg/m^3  orifice_area_max=1e-4 m^2  p_diff_orifice_area_TLU=0.2 : 0.2 : 1.2 MPa  p_gauge_orifice_area_TLU=0.2 : 0.2 : 1.2 MPa  orifice_area_TLU=[1e-10, 2e-05, 4e-05, 6e-05, 8e-05, .0001] m^2  Cd=0.64  leakage_fraction=1e-6  smoothing_factor=0.01  B_lam=0.999  area=pi*relief_vehTank_D^2/4 m^2
      settings: InternalSimscapePortConfiguration="{\"Bottom\":[],\"Left\":[{\"id\":\"A\",\"label\":\"A\",\"type\":\"foundation.gas.gas\"}],\"Right\":[{\"id\":\"B\",\"label\":\"B\",\"type\":\"foundation.gas.gas\"}],\"Top\":[]}"
  Reservoir (G) : fl_lib/Gas/Elements/Reservoir (G)  pressure_spec=foundation.enum.pressure_spec.atmospheric  reservoir_pressure=0.101325 MPa  reservoir_temperature=293.15 K  area_A=0.01 m^2
  Reservoir (G)1 : fl_lib/Gas/Elements/Reservoir (G)  pressure_spec=foundation.enum.pressure_spec.atmospheric  reservoir_pressure=0.101325 MPa  reservoir_temperature=T_env degC  area_A=pi*relief_vehTank_D^2/4 m^2
  Scope : Scope  NumInputPorts=3
  Tank : fl_lib/Gas/Elements/Constant Volume Chamber (G)  volume=V_vehTank l  num_ports=foundation.enum.num_ports.three  area_A=pi*inOut_vehTank_D^2/4 m^2  area_B=pi*relief_vehTank_D^2/4 m^2  area_C=pi*relief_vehTank_D^2 m^2  area_D=0.01 m^2  p_I_specify=on  p_I_priority=High  p_I=p_vehTank_init bar  p_I_nominal_specify=off  p_I_nominal_unit=MPa  p_I_nominal_value=1  T_I_specify=on  T_I_priority=High  T_I=T_Tank_init degC  T_I_nominal_specify=off  T_I_nominal_unit=K  T_I_nominal_value=1  rho_I_specify=off  rho_I_priority=None  rho_I=1.2 kg/m^3  rho_I_nominal_specify=off  rho_I_nominal_unit=kg/m^3  rho_I_nominal_value=1
      settings: InternalSimscapePortConfiguration="{\"Bottom\":[],\"Left\":[{\"id\":\"A\",\"label\":\"A\",\"type\":\"foundation.gas.gas\"},{\"id\":\"H\",\"label\":\"H\",\"type\":\"foundation.thermal.thermal\"}],\"Right\":[{\"id\":\"B\",\"label\":\"B\",\"type\":\"foundation.gas.gas\"},{\"id\":\"C\",\"label\":\"C\",\"type\":\"foundation.gas.gas\"}],\"Top\":[]}"
  Temperature Control Valve (G) : SimscapeFluids_lib/Gas/Valves & Orifices/Flow Control Valves/Temperature Control Valve (G)  valve_operation=fluids.gas.valves_orifices.flow_control_valves.enum.TemperatureValveOperation.Opens  temperature_sensing=fluids.gas.valves_orifices.flow_control_valves.enum.TemperatureValveSensing.ThermalPort  T_activation=TempCont_vehTank_setT degC  T_range=TempCont_vehTank_Trange deltadegC  tau=1.5 s  valve_parameterization=fluids.gas.valves_orifices.enum.OrificeParameterization.Cv  Cv_max=4  xT_Cv=0.7  Kv_max=3.6  xT_Kv=0.7  C_max=12 l/(bar*s)  B_crit_linear=0.3  m=0.5  T_ref_C=293.15 K  rho_ref_C=1.185 kg/m^3  orifice_area_max=1e-4 m^2  Cd=0.64  leakage_fraction=1e-6  smoothing_factor=0.01  B_lam=0.999  area=pi*TempCont_vehTank_D^2/4 m^2  T_sensor_specify=on  T_sensor_priority=High  T_sensor=T_Tank_init degC  T_sensor_nominal_specify=off  T_sensor_nominal_unit=K  T_sensor_nominal_value=1
      settings: InternalSimscapePortConfiguration="{\"Bottom\":[],\"Left\":[{\"id\":\"A\",\"label\":\"A\",\"type\":\"foundation.gas.gas\"}],\"Right\":[{\"id\":\"B\",\"label\":\"B\",\"type\":\"foundation.gas.gas\"}],\"Top\":[{\"id\":\"T_T\",\"label\":\"T\",\"type\":\"foundation.thermal.thermal\"}]}"
  Temperature Sensor : fl_lib/Thermal/Thermal Sensors/Temperature Sensor  temperature_measure=foundation.enum.MeasurementReference.difference
  Thermal Reference : fl_lib/Thermal/Thermal Elements/Thermal Reference
  Wall Mass : fl_lib/Thermal/Thermal Elements/Thermal Mass  mass_type=foundation.enum.constant_variable.constant  mass=M_vehTank kg  sp_heat=c_vehTank J/(K*kg)  mass_min=1e-6 kg  num_ports=foundation.enum.numPorts2.two  m_specify=off  m_priority=High  m=1 kg  m_nominal_specify=off  m_nominal_unit=kg  m_nominal_value=1  T_specify=on  T_priority=High  T=T_env degC  T_nominal_specify=off  T_nominal_unit=K  T_nominal_value=1  Q_specify=off  Q_priority=None  Q=0 W  Q_nominal_specify=off  Q_nominal_unit=W  Q_nominal_value=1
      settings: InternalSimscapePortConfiguration="{\"Bottom\":[],\"Left\":[{\"id\":\"M\",\"label\":\"\",\"type\":\"foundation.thermal.thermal\"}],\"Right\":[{\"id\":\"N\",\"label\":\"\",\"type\":\"foundation.thermal.thermal\"}],\"Top\":[]}"
  OTV : PMIOPort  Side=Left
  p_Tank : Outport
  T_Tank : Outport  Port=2
  m_Tank_In : Outport  Port=3
  wires:
  PS-Simulink Converter1/1 -> T_Tank/1, Scope/3  "T_Tank"
  PS-Simulink Converter/1 -> p_Tank/1, Scope/2  "p_Tank"
  PS-Simulink Converter2/1 -> Scope/1, Integrator/1, m_Tank_In/1  "m_Tank"
  Integrator/1 -> Display/1
  connections:
  PS-Simulink Converter1/LConn1 -- Temperature Sensor/RConn2
  Thermal Reference/LConn1 -- Temperature Sensor/RConn1
  Tank/LConn2 -- Temperature Control Valve (G)/LConn2 -- Temperature Sensor/LConn1 -- Internal Convection/LConn1
  Wall Mass/LConn1 -- Internal Convection/RConn1
  External Convection/LConn1 -- Wall Mass/RConn1
  Pressure & Temperature Sensor (G)/RConn1 -- PS-Simulink Converter/LConn1
  Mass & Energy Flow Rate Sensor (G)2/LConn1 -- OTV/RConn1
  Mass & Energy Flow Rate Sensor (G)2/RConn1 -- Pressure & Temperature Sensor (G)/LConn1 -- Tank/LConn1
  PS-Simulink Converter2/LConn1 -- Mass & Energy Flow Rate Sensor (G)2/RConn2
  Reservoir (G)/LConn1 -- Pressure Relief Valve (G)1/RConn1
  Tank/RConn1 -- Pressure Relief Valve (G)1/LConn1
  Environment Temperature/LConn1 -- External Convection/RConn1
  Temperature Control Valve (G)/RConn1 -- Reservoir (G)1/LConn1
  Temperature Control Valve (G)/LConn1 -- Tank/RConn2

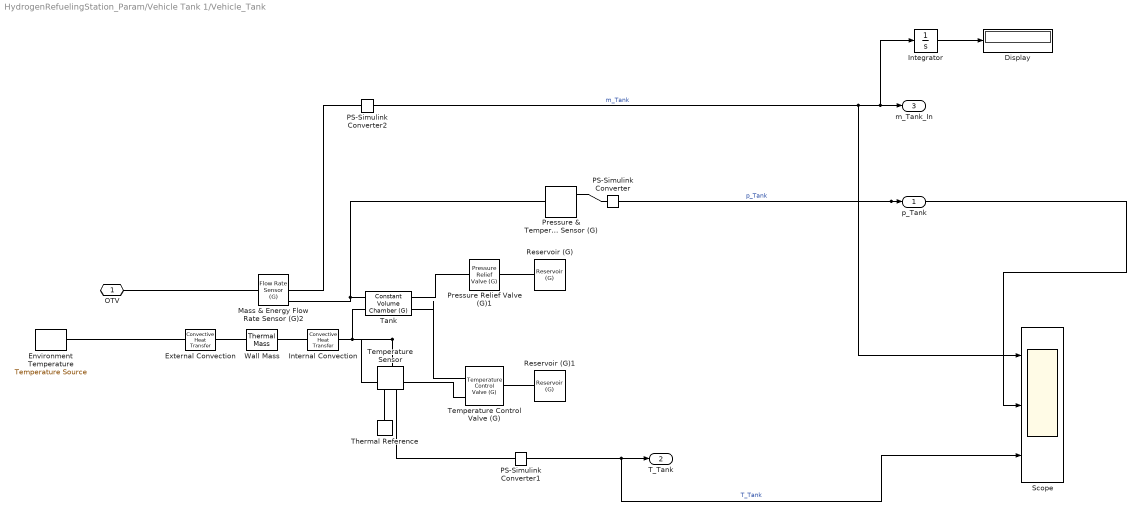
== system HydrogenRefuelingStation_Param/Vehicle Tank 1/Vehicle_Tank ==
  Display : Display
  Environment Temperature : fl_lib/Thermal/Thermal Sources/Temperature Source  temperature=T_env degC
  External Convection : fl_lib/Thermal/Thermal Elements/Convective Heat Transfer  thermal_type=foundation.enum.constant_variable.constant  area=2*pi*(ext_vehTank_D/2)*L_vehTank m^2  heat_tr_coeff=h_ext_vehTank W/(K*m^2)  min_heat_tr_coeff=1e-3 W/(K*m^2)  T_specify=off  T_priority=None  T=0 K  T_nominal_specify=off  T_nominal_unit=K  T_nominal_value=1  Q_specify=off  Q_priority=None  Q=0 W  Q_nominal_specify=off  Q_nominal_unit=W  Q_nominal_value=1
  Integrator : Integrator
  Internal Convection : fl_lib/Thermal/Thermal Elements/Convective Heat Transfer  thermal_type=foundation.enum.constant_variable.constant  area=2*pi*(int_vehTank_D/2)*L_vehTank m^2  heat_tr_coeff=h_int_vehTank W/(K*m^2)  min_heat_tr_coeff=1e-3 W/(K*m^2)  T_specify=off  T_priority=None  T=0 K  T_nominal_specify=off  T_nominal_unit=K  T_nominal_value=1  Q_specify=off  Q_priority=None  Q=0 W  Q_nominal_specify=off  Q_nominal_unit=W  Q_nominal_value=1
  Mass & Energy Flow Rate Sensor (G)2 : fl_lib/Gas/Sensors/Flow Rate Sensor (G)  mass_flow_measure=true  volumetric_flow_measure=false  volumetric_flow_conditions=foundation.enum.volumetric_flow_conditions.actual  p_std=0.101325 MPa  T_std=20 degC  energy_flow_measure=true
      settings: InternalSimscapePortConfiguration="{\"Bottom\":[{\"id\":\"PHI\",\"label\":\"φ\",\"type\":\"output\"}],\"Left\":[{\"id\":\"A\",\"label\":\"A\",\"type\":\"foundation.gas.gas\"}],\"Right\":[{\"id\":\"B\",\"label\":\"B\",\"type\":\"foundation.gas.gas\"},{\"id\":\"M\",\"label\":\"M\",\"type\":\"output\"}],\"Top\":[]}"
  PS-Simulink Converter : nesl_utility/PS-Simulink Converter  PhysicalDomain=network_engine_domain  SubClassName=ps_output  LeftPortType=input  RightPortType=output  PseudoPeriodic=off  Frequencies=[]  VectorFormat=inherit  Unit=bar  AffineConversion=off
  PS-Simulink Converter1 : nesl_utility/PS-Simulink Converter  PhysicalDomain=network_engine_domain  SubClassName=ps_output  LeftPortType=input  RightPortType=output  PseudoPeriodic=off  Frequencies=[]  VectorFormat=inherit  Unit=degC  AffineConversion=on
  PS-Simulink Converter2 : nesl_utility/PS-Simulink Converter  PhysicalDomain=network_engine_domain  SubClassName=ps_output  LeftPortType=input  RightPortType=output  PseudoPeriodic=off  Frequencies=[]  VectorFormat=inherit  Unit=kg/s  AffineConversion=off
  Pressure & Temperature Sensor (G) : fl_lib/Gas/Sensors/Pressure & Temperature Sensor (G)  reference=foundation.enum.MeasurementReference.absolute  pressure=true  pressure_spec=foundation.enum.PressureMeasementSpec.Absolute  temperature=true
      settings: InternalSimscapePortConfiguration="{\"Bottom\":[{\"id\":\"T\",\"label\":\"T\",\"type\":\"output\"}],\"Left\":[{\"id\":\"A\",\"label\":\"A\",\"type\":\"foundation.gas.gas\"}],\"Right\":[{\"id\":\"Pa\",\"label\":\"Pa\",\"type\":\"output\"}],\"Top\":[]}"
  Pressure Relief Valve (G)1 : SimscapeFluids_lib/Gas/Valves & Orifices/Pressure Control Valves/Pressure Relief Valve (G)  opening_pressure_spec=fluids.gas.valves_orifices.enum.PressureControlSpec.PressureA  valve_parameterization=fluids.gas.valves_orifices.enum.OrificeParameterization.Cv  opening_characteristic=fluids.gas.valves_orifices.enum.OpeningCharacteristics.Linear  p_set_differential=0 MPa  p_set_gauge=relief_vehTank_setP bar  p_range=relief_vehtank_range bar  Cv_max=4  p_diff_Cv_TLU=0.2 : 0.2 : 1.2 MPa  p_gauge_Cv_TLU=0.2 : 0.2 : 1.2 MPa  Cv_TLU=[1e-06, .8, 1.6, 2.4, 3.2, 4]  xT_Cv=0.7  Kv_max=3.6  p_diff_Kv_TLU=0.2 : 0.2 : 1.2 MPa  p_gauge_Kv_TLU=0.2 : 0.2 : 1.2 MPa  Kv_TLU=[1e-06, .72, 1.44, 2.16, 2.88, 3.6]  xT_Kv=0.7  C_max=12 l/(bar*s)  B_crit_linear=0.3  p_diff_C_TLU=0.2 : 0.2 : 1.2 MPa  p_gauge_C_TLU=0.2 : 0.2 : 1.2 MPa  C_TLU=[1e-05, 2.4, 4.8, 7.2, 9.6, 12] l/(bar*s)  B_crit_TLU=0.3 * ones(1, 6)  m=0.5  T_ref_C=293.15 K  rho_ref_C=1.185 kg/m^3  orifice_area_max=1e-4 m^2  p_diff_orifice_area_TLU=0.2 : 0.2 : 1.2 MPa  p_gauge_orifice_area_TLU=0.2 : 0.2 : 1.2 MPa  orifice_area_TLU=[1e-10, 2e-05, 4e-05, 6e-05, 8e-05, .0001] m^2  Cd=0.64  leakage_fraction=1e-6  smoothing_factor=0.01  B_lam=0.999  area=pi*relief_vehTank_D^2/4 m^2
      settings: InternalSimscapePortConfiguration="{\"Bottom\":[],\"Left\":[{\"id\":\"A\",\"label\":\"A\",\"type\":\"foundation.gas.gas\"}],\"Right\":[{\"id\":\"B\",\"label\":\"B\",\"type\":\"foundation.gas.gas\"}],\"Top\":[]}"
  Reservoir (G) : fl_lib/Gas/Elements/Reservoir (G)  pressure_spec=foundation.enum.pressure_spec.atmospheric  reservoir_pressure=0.101325 MPa  reservoir_temperature=293.15 K  area_A=0.01 m^2
  Reservoir (G)1 : fl_lib/Gas/Elements/Reservoir (G)  pressure_spec=foundation.enum.pressure_spec.atmospheric  reservoir_pressure=0.101325 MPa  reservoir_temperature=T_env degC  area_A=pi*relief_vehTank_D^2/4 m^2
  Scope : Scope  NumInputPorts=3
  Tank : fl_lib/Gas/Elements/Constant Volume Chamber (G)  volume=V_vehTank l  num_ports=foundation.enum.num_ports.three  area_A=pi*inOut_vehTank_D^2/4 m^2  area_B=pi*relief_vehTank_D^2/4 m^2  area_C=pi*relief_vehTank_D^2 m^2  area_D=0.01 m^2  p_I_specify=on  p_I_priority=High  p_I=p_vehTank_init bar  p_I_nominal_specify=off  p_I_nominal_unit=MPa  p_I_nominal_value=1  T_I_specify=on  T_I_priority=High  T_I=T_Tank_init degC  T_I_nominal_specify=off  T_I_nominal_unit=K  T_I_nominal_value=1  rho_I_specify=off  rho_I_priority=None  rho_I=1.2 kg/m^3  rho_I_nominal_specify=off  rho_I_nominal_unit=kg/m^3  rho_I_nominal_value=1
      settings: InternalSimscapePortConfiguration="{\"Bottom\":[],\"Left\":[{\"id\":\"A\",\"label\":\"A\",\"type\":\"foundation.gas.gas\"},{\"id\":\"H\",\"label\":\"H\",\"type\":\"foundation.thermal.thermal\"}],\"Right\":[{\"id\":\"B\",\"label\":\"B\",\"type\":\"foundation.gas.gas\"},{\"id\":\"C\",\"label\":\"C\",\"type\":\"foundation.gas.gas\"}],\"Top\":[]}"
  Temperature Control Valve (G) : SimscapeFluids_lib/Gas/Valves & Orifices/Flow Control Valves/Temperature Control Valve (G)  valve_operation=fluids.gas.valves_orifices.flow_control_valves.enum.TemperatureValveOperation.Opens  temperature_sensing=fluids.gas.valves_orifices.flow_control_valves.enum.TemperatureValveSensing.ThermalPort  T_activation=TempCont_vehTank_setT degC  T_range=TempCont_vehTank_Trange deltadegC  tau=1.5 s  valve_parameterization=fluids.gas.valves_orifices.enum.OrificeParameterization.Cv  Cv_max=4  xT_Cv=0.7  Kv_max=3.6  xT_Kv=0.7  C_max=12 l/(bar*s)  B_crit_linear=0.3  m=0.5  T_ref_C=293.15 K  rho_ref_C=1.185 kg/m^3  orifice_area_max=1e-4 m^2  Cd=0.64  leakage_fraction=1e-6  smoothing_factor=0.01  B_lam=0.999  area=pi*TempCont_vehTank_D^2/4 m^2  T_sensor_specify=off  T_sensor_priority=High  T_sensor=T_Tank_init degC  T_sensor_nominal_specify=off  T_sensor_nominal_unit=K  T_sensor_nominal_value=1
      settings: InternalSimscapePortConfiguration="{\"Bottom\":[],\"Left\":[{\"id\":\"A\",\"label\":\"A\",\"type\":\"foundation.gas.gas\"}],\"Right\":[{\"id\":\"B\",\"label\":\"B\",\"type\":\"foundation.gas.gas\"}],\"Top\":[{\"id\":\"T_T\",\"label\":\"T\",\"type\":\"foundation.thermal.thermal\"}]}"
  Temperature Sensor : fl_lib/Thermal/Thermal Sensors/Temperature Sensor  temperature_measure=foundation.enum.MeasurementReference.difference
  Thermal Reference : fl_lib/Thermal/Thermal Elements/Thermal Reference
  Wall Mass : fl_lib/Thermal/Thermal Elements/Thermal Mass  mass_type=foundation.enum.constant_variable.constant  mass=M_vehTank kg  sp_heat=c_vehTank J/(K*kg)  mass_min=1e-6 kg  num_ports=foundation.enum.numPorts2.two  m_specify=off  m_priority=High  m=1 kg  m_nominal_specify=off  m_nominal_unit=kg  m_nominal_value=1  T_specify=on  T_priority=High  T=T_env degC  T_nominal_specify=off  T_nominal_unit=K  T_nominal_value=1  Q_specify=off  Q_priority=None  Q=0 W  Q_nominal_specify=off  Q_nominal_unit=W  Q_nominal_value=1
      settings: InternalSimscapePortConfiguration="{\"Bottom\":[],\"Left\":[{\"id\":\"M\",\"label\":\"\",\"type\":\"foundation.thermal.thermal\"}],\"Right\":[{\"id\":\"N\",\"label\":\"\",\"type\":\"foundation.thermal.thermal\"}],\"Top\":[]}"
  OTV : PMIOPort  Side=Left
  p_Tank : Outport
  T_Tank : Outport  Port=2
  m_Tank_In : Outport  Port=3
  wires:
  Integrator/1 -> Display/1
  PS-Simulink Converter2/1 -> m_Tank_In/1, Integrator/1, Scope/1  "m_Tank"
  PS-Simulink Converter/1 -> Scope/2, p_Tank/1  "p_Tank"
  PS-Simulink Converter1/1 -> Scope/3, T_Tank/1  "T_Tank"
  connections:
  Temperature Control Valve (G)/LConn1 -- Tank/RConn2
  Temperature Control Valve (G)/RConn1 -- Reservoir (G)1/LConn1
  Environment Temperature/LConn1 -- External Convection/RConn1
  Tank/RConn1 -- Pressure Relief Valve (G)1/LConn1
  Reservoir (G)/LConn1 -- Pressure Relief Valve (G)1/RConn1
  PS-Simulink Converter2/LConn1 -- Mass & Energy Flow Rate Sensor (G)2/RConn2
  Tank/LConn1 -- Pressure & Temperature Sensor (G)/LConn1 -- Mass & Energy Flow Rate Sensor (G)2/RConn1
  Mass & Energy Flow Rate Sensor (G)2/LConn1 -- OTV/RConn1
  Pressure & Temperature Sensor (G)/RConn1 -- PS-Simulink Converter/LConn1
  External Convection/LConn1 -- Wall Mass/RConn1
  Wall Mass/LConn1 -- Internal Convection/RConn1
  Internal Convection/LConn1 -- Temperature Sensor/LConn1 -- Temperature Control Valve (G)/LConn2 -- Tank/LConn2
  Thermal Reference/LConn1 -- Temperature Sensor/RConn1
  PS-Simulink Converter1/LConn1 -- Temperature Sensor/RConn2
